simulink model "speed_modelo_motor"  (R2022b)
settings: Solver=VariableStepAuto  StartTime=0.0  StopTime=4  FixedStep=0.01  MaxStep=0.00005  RelTol=1e-3
values from neighbouring files (symbols this model uses):
  frecuencia = (3:3:48)    [carga_datos_slip11.m]
  FuerzaXslip = [-AuxX(1:end-1,:,:);FuerzaX(1:end,:,:)]    [carga_datos_slip11.m]
  Ipeak = (10:10:100)    [carga_datos_slip11.m]
  L = zeros((length(current)-2), length(slip),length(frecuencia))    [carga_datos_slip11.m]
  mass = 200    [carga_datos_slip11.m]
  pole_length = 0.114    [carga_datos_slip11.m]
  r = 0.384    [carga_datos_slip11.m]
  slip = (0:0.1:1)    [carga_datos_slip11.m]
  slipFuerza = (-1:0.1:1)    [carga_datos_slip11.m]
  vel_motor_max_f = []    [carga_datos_slip11.m]
undefined symbols (not defined in the file or in its folder): frec_max_f
libraries: slpidlib x2, eePowerMeasurement x1
settings Model: Creator=mique  LastModifiedBy=mique
settings SolverCC: ZeroCrossAlgorithm=Adaptive
settings DebuggingCC: IgnoredZcDiagnostic=none

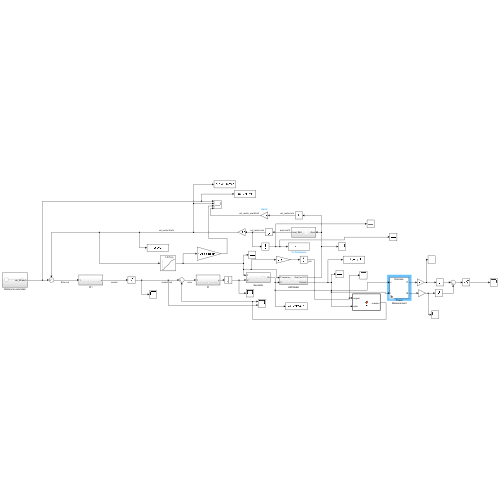
[thumbnail: Simulink's stored preview of the top-level diagram]
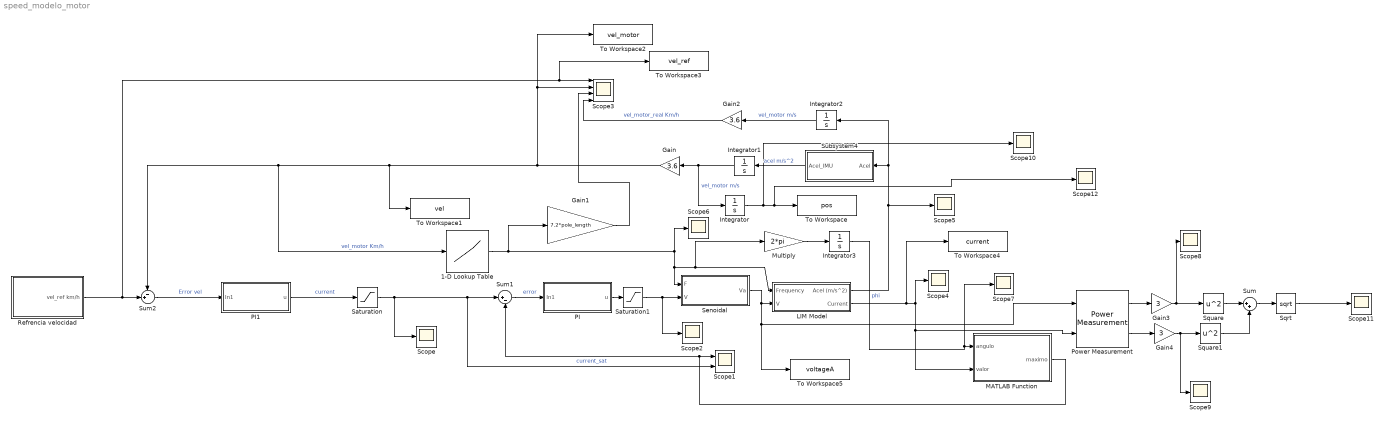
== system speed_modelo_motor ==
  1-D Lookup Table : Lookup_n-D  NumberOfTableDimensions=1  BreakpointsForDimension1=vel_motor_max_f  Table=frec_max_f  InternalRulePriority=Speed  RndMeth=Simplest
  Gain : Gain  Gain=3.6
  Gain1 : Gain  Gain=7.2*pole_length
  Gain2 : Gain  Gain=3.6
  Gain3 : Gain  Gain=3
  Gain4 : Gain  Gain=3
  Integrator : Integrator
  Integrator1 : Integrator
  Integrator2 : Integrator
  Integrator3 : Integrator  WrappedStateUpperValue=2*pi  WrappedStateLowerValue=0
  LIM Model : Subsystem
  MATLAB Function : MATLAB Function  TreatAsAtomicUnit=on
  Multiply : Gain  Gain=2*pi
  PI : Subsystem
  PI1 : Subsystem
  Power Measurement : eePowerMeasurement/Power Measurement  LabelModeActiveChoice=Discrete  F=8  K=[0 1 2 3 4]  Ts=0.0002
  Refrencia velocidad : Subsystem
  Saturation : Saturate  UpperLimit=100  LowerLimit=-100
  Saturation1 : Saturate  UpperLimit=200  LowerLimit=-200
  Scope{,2,4..12} (11 alike) : Scope
  Scope1 : Scope  NumInputPorts=2
  Scope3 : Scope  NumInputPorts=4
  Senoidal : Subsystem
  Sqrt : Sqrt
  Square : Math  Operator=square
  Square1 : Math  Operator=square
  Subsystem4 : Subsystem
  Sum : Sum  Inputs=|++
  Sum1 : Sum  Inputs=|+-
  Sum2 : Sum  Inputs=-+|
  To Workspace : ToWorkspace  VariableName=pos  SampleTime=-1
  To Workspace1 : ToWorkspace  VariableName=vel  SampleTime=-1
  To Workspace2 : ToWorkspace  VariableName=vel_motor  SampleTime=-1
  To Workspace3 : ToWorkspace  VariableName=vel_ref  SampleTime=-1
  To Workspace4 : ToWorkspace  VariableName=current  SampleTime=-1
  To Workspace5 : ToWorkspace  VariableName=voltageA  SaveFormat=Timeseries  SampleTime=-1
  wires:
  Integrator1/1 -> Integrator/1, Gain/1  "vel_motor m/s"
  Gain/1 -> To Workspace2/1, Scope3/2, To Workspace1/1, Sum2/1, 1-D Lookup Table/1  "vel_motor Km/h"
  LIM Model/1(Acel (m/s^2)) -> Integrator2/1, Subsystem4/1(Acel), Scope5/1
  Integrator/1 -> Scope10/1, Scope12/1, To Workspace/1
  PI/1(u) -> Saturation1/1
  Sum1/1 -> PI/1(In1)  "error"
  Sum2/1 -> PI1/1(In1)  "Error vel"
  Refrencia velocidad/1(vel_ref km/h) -> To Workspace3/1, Scope3/1, Sum2/2
  PI1/1(u) -> Saturation/1  "current"
  Gain1/1 -> Scope3/3
  Saturation/1 -> Scope/1, Scope1/2, Sum1/1  "current_sat"
  Subsystem4/1(Acel_IMU) -> Integrator1/1  "acel m/s^2"
  Integrator2/1 -> Gain2/1  "vel_motor m/s"
  Gain2/1 -> Scope3/4  "vel_motor_real Km/h"
  1-D Lookup Table/1 -> Scope6/1, Senoidal/1(F), LIM Model/1(Frequency), Multiply/1, Gain1/1
  MATLAB Function/1(maximo) -> Sum1/2, Scope1/1
  LIM Model/2(Current) -> To Workspace4/1, Scope4/1, MATLAB Function/2(valor), Power Measurement/2
  Multiply/1 -> Integrator3/1
  Integrator3/1 -> Scope7/1, MATLAB Function/1(angulo)  "phi"
  Senoidal/1(Va) -> To Workspace5/1, Power Measurement/1, LIM Model/2("V ")
  Power Measurement/1 -> Gain3/1
  Gain3/1 -> Square/1, Scope8/1
  Power Measurement/2 -> Gain4/1
  Gain4/1 -> Scope9/1, Square1/1
  Saturation1/1 -> Senoidal/2(V), Scope2/1
  Square/1 -> Sum/1
  Square1/1 -> Sum/2
  Sum/1 -> Sqrt/1
  Sqrt/1 -> Scope11/1

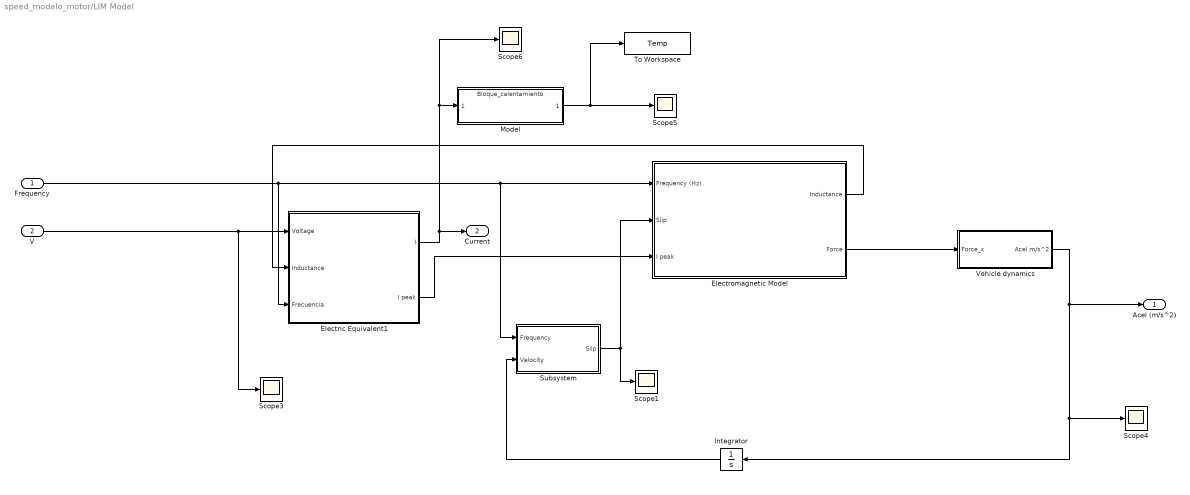
== system speed_modelo_motor/LIM Model ==
  Frequency : Inport
  "V " : Inport  Port=2
  Electric Equivalent1 : Subsystem
  Electromagnetic Model : Subsystem
  Integrator : Integrator
  Model : ModelReference  ModelNameDialog=Bloque_calentamiento.slx  SimulationMode=Normal  ModelReferenceVersion=3.6
  Scope{1,3..6} (5 alike) : Scope
  Subsystem : Subsystem
  To Workspace : ToWorkspace  VariableName=Temp  SampleTime=-1
  Vehicle dynamics : Subsystem
  Acel (m/s^2) : Outport
  Current : Outport  Port=2
  wires:
  Subsystem/1(Slip) -> Scope1/1, Electromagnetic Model/2(Slip)
  Vehicle dynamics/1(Acel m/s^2) -> Integrator/1, Scope4/1, Acel (m/s^2)/1
  Electric Equivalent1/2(I peak) -> Electromagnetic Model/3(I peak)
  Electromagnetic Model/1(Inductance) -> Electric Equivalent1/2(Inductance)
  Frequency/1 -> Electric Equivalent1/3(Frecuencia), Subsystem/1(Frequency), Electromagnetic Model/1(Frequency (Hz))
  Integrator/1 -> Subsystem/2(Velocity)
  "V "/1 -> Scope3/1, Electric Equivalent1/1(Voltage)
  Electric Equivalent1/1("I ") -> Current/1, Scope6/1, Model/1
  Model/1 -> To Workspace/1, Scope5/1
  Electromagnetic Model/2(Force) -> Vehicle dynamics/1(Force_x)

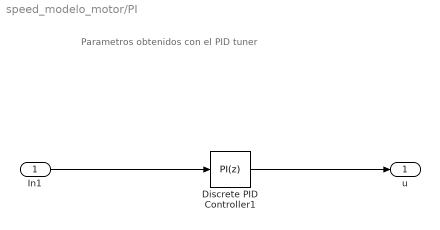
== system speed_modelo_motor/PI ==
  note: Parametros obtenidos con el PID tuner
  In1 : Inport
  Discrete PID Controller1 : slpidlib/PID Controller  Controller=PI  Form=Parallel  TimeDomain=Discrete-time  UseExternalTs=off  SampleTime=0.0002  IntegratorMethod=Forward Euler  FilterMethod=Forward Euler  ControllerParametersSource=internal  P=0.2  I=5  UseKiTs=off  D=0.5  N=10  UseFilter=on  TunerSelectOption=Transfer Function Based (PID Tuner App)  InitialConditionSource=internal  InitialConditionForIntegrator=0  InitialConditionForFilter=0  DifferentiatorICPrevScaledInput=0  ExternalReset=none  TrackingMode=off  Kt=1  LimitOutput=off  SatLimitsSource=internal  UpperSaturationLimit=100  LowerSaturationLimit=-inf  LinearizeAsGain=off  AntiWindupMode=back-calculation  Kb=1  LimitIntegrator=off  UpperIntegratorSaturationLimit=15  LowerIntegratorSaturationLimit=-15  POutMin=[]  POutMax=[]  IOutMin=[]  IOutMax=[]  DOutMin=[]  DOutMax=[]  NOutMin=[]  NOutMax=[]  SumOutMin=[]  SumOutMax=[]  SaturationOutMin=[]  SaturationOutMax=[]  PParamMin=[]  PParamMax=[]  IParamMin=[]  IParamMax=[]  DParamMin=[]  DParamMax=[]  NParamMin=[]  NParamMax=[]  KbParamMin=[]  KbParamMax=[]  KtParamMin=[]  KtParamMax=[]  KbOutMin=[]  KbOutMax=[]  KtOutMin=[]  KtOutMax=[]  IntegratorOutMin=[]  IntegratorOutMax=[]  FilterOutMin=[]  FilterOutMax=[]  SumI1OutMin=[]  SumI1OutMax=[]  SumI2OutMin=[]  SumI2OutMax=[]  SumI3OutMin=[]  SumI3OutMax=[]  SumI4OutMin=[]  SumI4OutMax=[]  SumDOutMin=[]  SumDOutMax=[]  DifferentiatorOutMin=[]  DifferentiatorOutMax=[]  FilterDiffOutCoefMin=[]  FilterDiffOutCoefMax=[]  ReciprocalOutMin=[]  ReciprocalOutMax=[]  SumDenOutMin=[]  SumDenOutMax=[]  SumNumOutMin=[]  SumNumOutMax=[]  DivideOutMin=[]  DivideOutMax=[]  UdiffTsProdOutMin=[]  UdiffTsProdOutMax=[]  NTsProdOutMin=[]  NTsProdOutMax=[]  UintegralTsProdOutMin=[]  UintegralTsProdOutMax=[]  UngainTsProdOutMin=[]  UngainTsProdOutMax=[]  ClampingZeroOutDataTypeStr=Inherit: Inherit via back propagation  ClampingZeroOutMin=[]  ClampingZeroOutMax=[]  FilterDenConstantOutDataTypeStr=Inherit: Inherit via back propagation  FilterDenConstantOutMin=[]  FilterDenConstantOutMax=[]  PCopyOutDataTypeStr=Inherit: Inherit via back propagation  PCopyOutMin=[]  PCopyOutMax=[]  NCopyOutDataTypeStr=Inherit: Inherit via back propagation  NCopyOutMin=[]  NCopyOutMax=[]  IntegratorContinuousStateAttributes=''  IntegratorStateMustResolveToSignalObject=off  IntegratorRTWStateStorageClass=Auto  FilterContinuousStateAttributes=''  FilterStateMustResolveToSignalObject=off  FilterRTWStateStorageClass=Auto  ParallelPVariant=InternalParameters  IdealPVariant=Disabled  IVariant=InternalParameters  DVariant=Disabled  IntegratorVariant=Discrete  SatVariant=Disabled  AWVariant=Passthrough  PCopyVariant=Disabled  TRVariant=Disabled  FdbkBlocksVariant=Forward  IdealPFdbkVariant=Disabled  SatFdbkVariant=Disabled  DerivativeFilterVariant=Disabled  NVariant=Disabled  NCopyVariant=Disabled_SignalSpec  FilterICVariant=Disabled  IntegratorICVariant=InternalICs  ExternalResetVariant=Disabled  TRSumVariant=Passthrough  SumFdbkVariant=Disabled  SumVariant=Sum_PI  TsampFilterVariant=InternalTs  TsampNgainVariant=Passthrough  TsampIntegralVariant=Passthrough  ExternalSaturationOutDataTypeStr=Inherit: Same as second input
      settings: LibrarySourceBlock=simulink/Discrete/Discrete PID Controller
  u : Outport
  wires:
  In1/1 -> Discrete PID Controller1/1
  Discrete PID Controller1/1 -> u/1

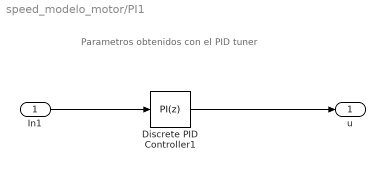
== system speed_modelo_motor/PI1 ==
  note: Parametros obtenidos con el PID tuner
  In1 : Inport
  Discrete PID Controller1 : slpidlib/PID Controller  Controller=PI  Form=Parallel  TimeDomain=Discrete-time  UseExternalTs=off  SampleTime=0.001  IntegratorMethod=Forward Euler  FilterMethod=Forward Euler  ControllerParametersSource=internal  P=25  I=18  UseKiTs=off  D=0.2  N=10  UseFilter=on  TunerSelectOption=Transfer Function Based (PID Tuner App)  InitialConditionSource=internal  InitialConditionForIntegrator=0  InitialConditionForFilter=0  DifferentiatorICPrevScaledInput=0  ExternalReset=none  TrackingMode=off  Kt=1  LimitOutput=off  SatLimitsSource=internal  UpperSaturationLimit=10  LowerSaturationLimit=-inf  LinearizeAsGain=off  AntiWindupMode=back-calculation  Kb=1  LimitIntegrator=on  UpperIntegratorSaturationLimit=15  LowerIntegratorSaturationLimit=-15  POutMin=[]  POutMax=[]  IOutMin=[]  IOutMax=[]  DOutMin=[]  DOutMax=[]  NOutMin=[]  NOutMax=[]  SumOutMin=[]  SumOutMax=[]  SaturationOutMin=[]  SaturationOutMax=[]  PParamMin=[]  PParamMax=[]  IParamMin=[]  IParamMax=[]  DParamMin=[]  DParamMax=[]  NParamMin=[]  NParamMax=[]  KbParamMin=[]  KbParamMax=[]  KtParamMin=[]  KtParamMax=[]  KbOutMin=[]  KbOutMax=[]  KtOutMin=[]  KtOutMax=[]  IntegratorOutMin=[]  IntegratorOutMax=[]  FilterOutMin=[]  FilterOutMax=[]  SumI1OutMin=[]  SumI1OutMax=[]  SumI2OutMin=[]  SumI2OutMax=[]  SumI3OutMin=[]  SumI3OutMax=[]  SumI4OutMin=[]  SumI4OutMax=[]  SumDOutMin=[]  SumDOutMax=[]  DifferentiatorOutMin=[]  DifferentiatorOutMax=[]  FilterDiffOutCoefMin=[]  FilterDiffOutCoefMax=[]  ReciprocalOutMin=[]  ReciprocalOutMax=[]  SumDenOutMin=[]  SumDenOutMax=[]  SumNumOutMin=[]  SumNumOutMax=[]  DivideOutMin=[]  DivideOutMax=[]  UdiffTsProdOutMin=[]  UdiffTsProdOutMax=[]  NTsProdOutMin=[]  NTsProdOutMax=[]  UintegralTsProdOutMin=[]  UintegralTsProdOutMax=[]  UngainTsProdOutMin=[]  UngainTsProdOutMax=[]  ClampingZeroOutDataTypeStr=Inherit: Inherit via back propagation  ClampingZeroOutMin=[]  ClampingZeroOutMax=[]  FilterDenConstantOutDataTypeStr=Inherit: Inherit via back propagation  FilterDenConstantOutMin=[]  FilterDenConstantOutMax=[]  PCopyOutDataTypeStr=Inherit: Inherit via back propagation  PCopyOutMin=[]  PCopyOutMax=[]  NCopyOutDataTypeStr=Inherit: Inherit via back propagation  NCopyOutMin=[]  NCopyOutMax=[]  IntegratorContinuousStateAttributes=''  IntegratorStateMustResolveToSignalObject=off  IntegratorRTWStateStorageClass=Auto  FilterContinuousStateAttributes=''  FilterStateMustResolveToSignalObject=off  FilterRTWStateStorageClass=Auto  ParallelPVariant=InternalParameters  IdealPVariant=Disabled  IVariant=InternalParameters  DVariant=Disabled  IntegratorVariant=Discrete  SatVariant=Disabled  AWVariant=Passthrough  PCopyVariant=Disabled  TRVariant=Disabled  FdbkBlocksVariant=Forward  IdealPFdbkVariant=Disabled  SatFdbkVariant=Disabled  DerivativeFilterVariant=Disabled  NVariant=Disabled  NCopyVariant=Disabled_SignalSpec  FilterICVariant=Disabled  IntegratorICVariant=InternalICs  ExternalResetVariant=Disabled  TRSumVariant=Passthrough  SumFdbkVariant=Disabled  SumVariant=Sum_PI  TsampFilterVariant=InternalTs  TsampNgainVariant=Passthrough  TsampIntegralVariant=Passthrough  ExternalSaturationOutDataTypeStr=Inherit: Same as second input
      settings: LibrarySourceBlock=simulink/Discrete/Discrete PID Controller
  u : Outport
  wires:
  Discrete PID Controller1/1 -> u/1
  In1/1 -> Discrete PID Controller1/1

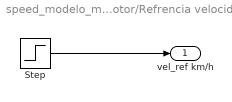
== system speed_modelo_motor/Refrencia velocidad ==
  Step : Step  Time=0.5  After=35  SampleTime=0
  vel_ref km/h : Outport
  wires:
  Step/1 -> vel_ref km/h/1

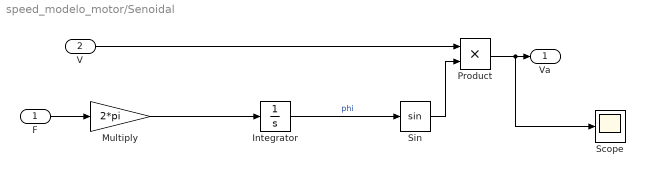
== system speed_modelo_motor/Senoidal ==
  F : Inport
  V : Inport  Port=2
  Integrator : Integrator  WrapState=on  WrappedStateUpperValue=2*pi  WrappedStateLowerValue=0
  Multiply : Gain  Gain=2*pi
  Product : Product
  Scope : Scope
  Sin : Trigonometry
  Va : Outport
  wires:
  Integrator/1 -> Sin/1  "phi"
  V/1 -> Product/1
  Sin/1 -> Product/2
  Product/1 -> Scope/1, Va/1
  F/1 -> Multiply/1
  Multiply/1 -> Integrator/1

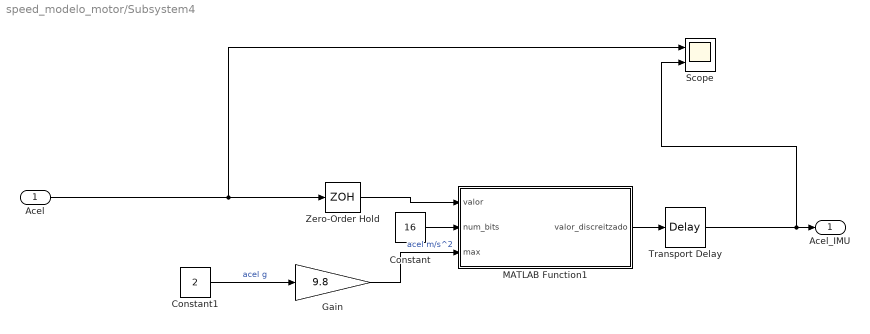
== system speed_modelo_motor/Subsystem4 ==
  Acel : Inport
  Constant : Constant  Value=16
  Constant1 : Constant  Value=2
  Gain : Gain  Gain=9.8
  MATLAB Function1 : MATLAB Function  TreatAsAtomicUnit=on
  Scope : Scope  NumInputPorts=2
  Transport Delay : TransportDelay  DelayTime=0.001
  Zero-Order Hold : ZeroOrderHold  SampleTime=0.001
  Acel_IMU : Outport
  wires:
  MATLAB Function1/1(valor_discreitzado) -> Transport Delay/1
  Zero-Order Hold/1 -> MATLAB Function1/1(valor)
  Constant1/1 -> Gain/1  "acel g"
  Constant/1 -> MATLAB Function1/2(num_bits)
  Gain/1 -> MATLAB Function1/3(max)  "acel m/s^2"
  Transport Delay/1 -> Scope/2, Acel_IMU/1
  Acel/1 -> Scope/1, Zero-Order Hold/1

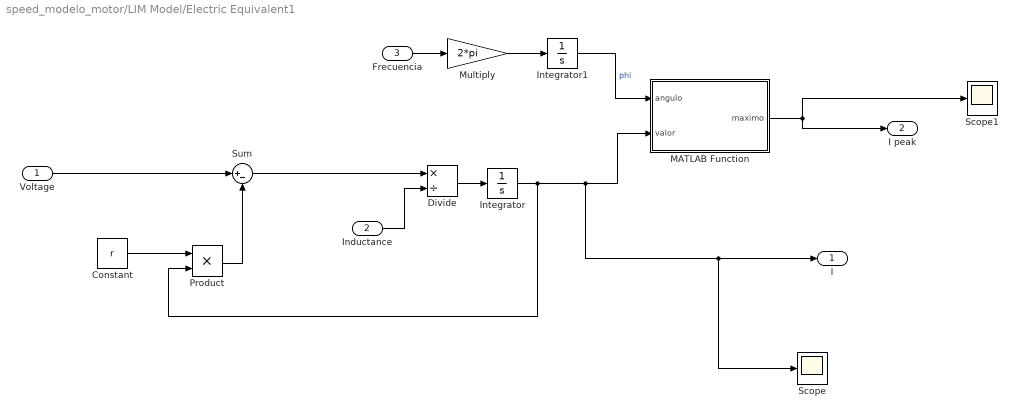
== system speed_modelo_motor/LIM Model/Electric Equivalent1 ==
  Voltage : Inport
  Inductance : Inport  Port=2
  Frecuencia : Inport  Port=3
  Constant : Constant  Value=r
  Divide : Product  Inputs=*/
  Integrator : Integrator
  Integrator1 : Integrator  WrappedStateUpperValue=2*pi  WrappedStateLowerValue=0
  MATLAB Function : MATLAB Function  TreatAsAtomicUnit=on
  Multiply : Gain  Gain=2*pi
  Product : Product
  Scope : Scope
  Scope1 : Scope
  Sum : Sum  Inputs=|+-
  "I " : Outport
  I peak : Outport  Port=2
  wires:
  Voltage/1 -> Sum/1
  Integrator/1 -> Scope/1, "I "/1, MATLAB Function/2(valor), Product/2
  Constant/1 -> Product/1
  Product/1 -> Sum/2
  Divide/1 -> Integrator/1
  Sum/1 -> Divide/1
  Inductance/1 -> Divide/2
  MATLAB Function/1(maximo) -> I peak/1, Scope1/1
  Multiply/1 -> Integrator1/1
  Frecuencia/1 -> Multiply/1
  Integrator1/1 -> MATLAB Function/1(angulo)  "phi"

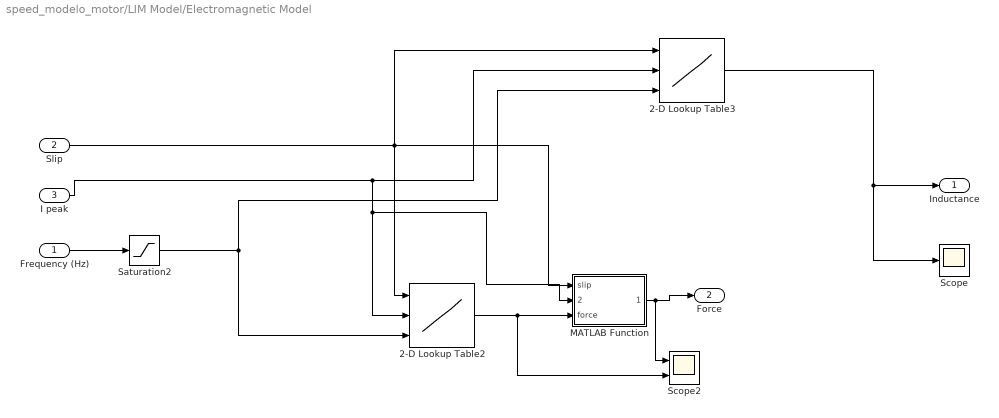
== system speed_modelo_motor/LIM Model/Electromagnetic Model ==
  Frequency (Hz) : Inport
  Slip : Inport  Port=2
  I peak : Inport  Port=3
  2-D Lookup Table2 : Lookup_n-D  NumberOfTableDimensions=3  BreakpointsForDimension1=slipFuerza  BreakpointsForDimension2=Ipeak  BreakpointsForDimension3=frecuencia  Table=FuerzaXslip  InternalRulePriority=Speed  RndMeth=Simplest
      settings: InputPortMap=u0,u1,u2
  2-D Lookup Table3 : Lookup_n-D  NumberOfTableDimensions=3  BreakpointsForDimension1=Ipeak(2:(end-1))  BreakpointsForDimension2=slip  BreakpointsForDimension3=frecuencia  Table=L  InterpMethod=Nearest  InternalRulePriority=Speed  RndMeth=Simplest
      settings: InputPortMap=u0,u1,u2
  MATLAB Function : MATLAB Function  TreatAsAtomicUnit=on
  Saturation2 : Saturate  UpperLimit=48  LowerLimit=3
  Scope : Scope
  Scope2 : Scope  NumInputPorts=2
  Inductance : Outport
  Force : Outport  Port=2
  wires:
  Frequency (Hz)/1 -> Saturation2/1
  2-D Lookup Table3/1 -> Scope/1, Inductance/1
  Saturation2/1 -> 2-D Lookup Table2/3, 2-D Lookup Table3/3
  MATLAB Function/1(fuerza_real) -> Scope2/1, Force/1
  I peak/1 -> MATLAB Function/2(current), 2-D Lookup Table2/2, 2-D Lookup Table3/2
  Slip/1 -> MATLAB Function/1(slip), 2-D Lookup Table2/1, 2-D Lookup Table3/1
  2-D Lookup Table2/1 -> Scope2/2, MATLAB Function/3(force)

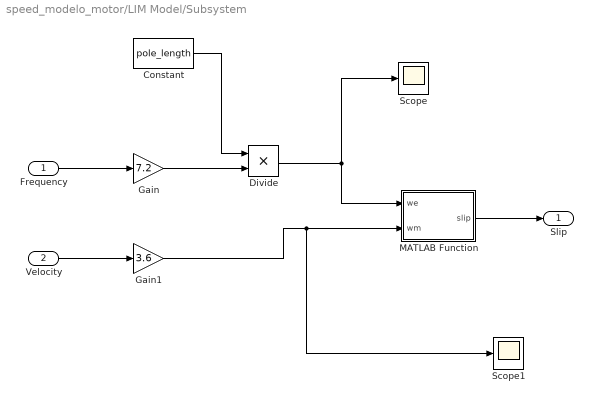
== system speed_modelo_motor/LIM Model/Subsystem ==
  Frequency : Inport
  Velocity : Inport  Port=2
  Constant : Constant  Value=pole_length
  Divide : Product  Inputs=**
  Gain : Gain  Gain=7.2
  Gain1 : Gain  Gain=3.6
  MATLAB Function : MATLAB Function  TreatAsAtomicUnit=on
  Scope : Scope
  Scope1 : Scope
  Slip : Outport
  wires:
  Frequency/1 -> Gain/1
  MATLAB Function/1(slip) -> Slip/1
  Gain/1 -> Divide/2
  Constant/1 -> Divide/1
  Divide/1 -> Scope/1, MATLAB Function/1(we)
  Velocity/1 -> Gain1/1
  Gain1/1 -> Scope1/1, MATLAB Function/2(wm)

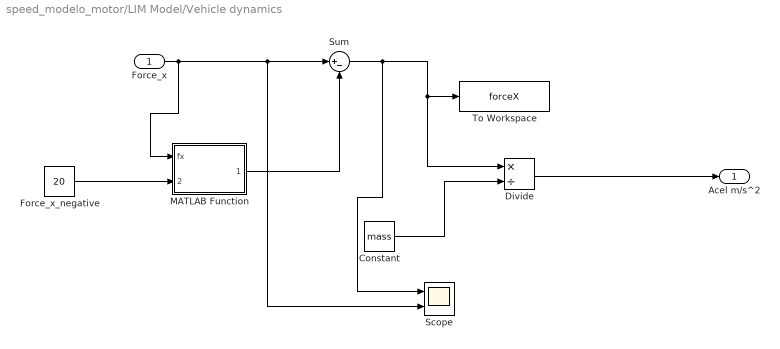
== system speed_modelo_motor/LIM Model/Vehicle dynamics ==
  Force_x : Inport
  Constant : Constant  Value=mass
  Divide : Product  Inputs=*/
  Force_x_negative : Constant  Value=20
  MATLAB Function : MATLAB Function  TreatAsAtomicUnit=on
  Scope : Scope  NumInputPorts=2
  Sum : Sum  Inputs=|+-
  To Workspace : ToWorkspace  VariableName=forceX  SampleTime=-1
  Acel m/s^2 : Outport
  wires:
  Divide/1 -> Acel m/s^2/1
  Constant/1 -> Divide/2
  Force_x/1 -> MATLAB Function/1(fx), Scope/2, Sum/1
  Sum/1 -> Scope/1, Divide/1, To Workspace/1
  Force_x_negative/1 -> MATLAB Function/2(fx_Contra)
  MATLAB Function/1(fx_contraReal) -> Sum/2

== matlab function speed_modelo_motor/LIM Model/Electromagnetic Model/MATLAB Function ==
  data: slip input; fuerza_real output; current input; force input
function fuerza_real = fcn(slip,current,force)


if slip == 0 || current== 0

    fuerza_real=0;

elseif slip<0 
    fuerza_real=-abs(force);
else
    fuerza_real=force;
end

== matlab function speed_modelo_motor/LIM Model/Vehicle dynamics/MATLAB Function ==
  data: fx input; fx_contraReal output; fx_Contra input
function fx_contraReal = fcn(fx,fx_Contra)


if fx>fx_Contra
    fx_contraReal=fx_Contra;
else
    fx_contraReal=fx;
end

== matlab function speed_modelo_motor/LIM Model/Electric Equivalent1/MATLAB Function ==
  settings: updateMethod=DISCRETE
  data: angulo input; maximo output; valor input
function maximo = fcn(angulo,valor)

   persistent antiguo_maximo
    if isempty(antiguo_maximo)
       antiguo_maximo=0;
    end
    persistent angulo_maximo
    if isempty(angulo_maximo)
       angulo_maximo=0;
    end


if valor>=antiguo_maximo
    maximo=valor;
    antiguo_maximo=valor;
    angulo_maximo=angulo;
else
    maximo=antiguo_maximo;
    if angulo>angulo_maximo+4*pi
        maximo=valor;
        antiguo_maximo=valor;
        angulo_maximo=angulo;
    end
    
end

== matlab function speed_modelo_motor/LIM Model/Subsystem/MATLAB Function ==
  data: we input; slip output; wm input
function slip = fcn(we,wm)

slip = (we-wm)/we;

== matlab function speed_modelo_motor/MATLAB Function ==
  settings: updateMethod=DISCRETE
  data: angulo input; maximo output; valor input
function maximo = fcn(angulo,valor)

   persistent antiguo_maximo
    if isempty(antiguo_maximo)
       antiguo_maximo=0;
    end
    persistent angulo_maximo
    if isempty(angulo_maximo)
       angulo_maximo=0;
    end


if valor>=antiguo_maximo
    maximo=valor;
    antiguo_maximo=valor;
    angulo_maximo=angulo;
else
    maximo=antiguo_maximo;
    if angulo>angulo_maximo+4*pi
        maximo=valor;
        antiguo_maximo=valor;
        angulo_maximo=angulo;
    end
    
end

== matlab function speed_modelo_motor/Subsystem4/MATLAB Function1 ==
  data: valor input; valor_discreitzado output; num_bits input; max input
function valor_discreitzado  = fcn(valor,num_bits,max)

min=-max;
num_valores=2^num_bits;
if(valor>max)
    valor_discreitzado=max;
    return
end
if(valor<min)
    valor_discreitzado=min;
    return
end


valor_escalon=(max-min)/(num_valores-1);


i=min;
 while(i<max)
    if(i+valor_escalon/2>valor)
        valor_discreitzado=i;
        return
    end
    i=i+valor_escalon;
end



      valor_discreitzado=max;
end
